simulink subsystem "Motor"  (R2024a)
settings: Solver=VariableStepAuto  StartTime=0.0  StopTime=10.0  RelTol=1e-3
values from neighbouring files (symbols this model uses):
  useGenerator = Simulink.Parameter    [LAFES_saveas.m]
settings Model: Creator=20192648  LastModifiedBy=20192648
settings ConfigComp: CovBoundaryAbsTol=1.0e-5

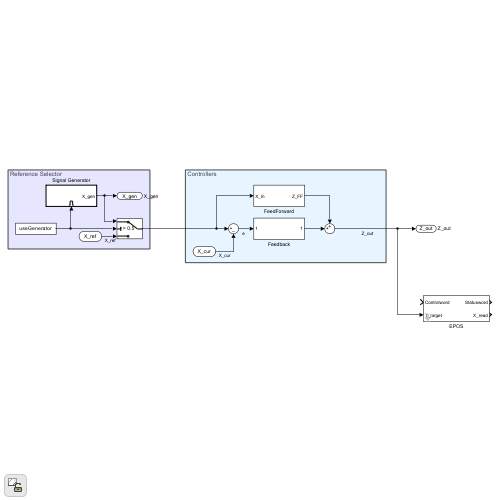
[thumbnail: Simulink's stored preview of the top-level diagram]
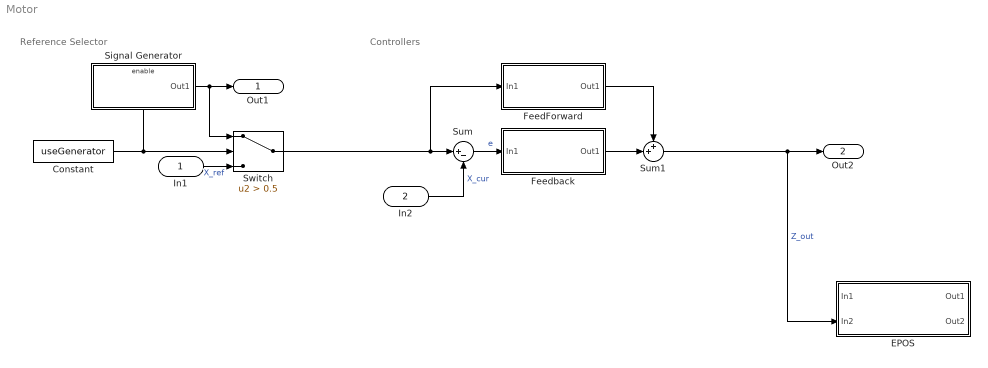
== system Motor ==
  note: Controllers
  note: Reference Selector
  In1 : Inport
  In2 : Inport  Port=2
  Constant : Constant  Value=useGenerator
  EPOS : Subsystem  mask{link_id=1, operating_mode=CyclicSynchronousTorque}
      mask prompts: link_id "link id > 0"; operating_mode "Operating mode of the drive"
      mask TypeOptions operating_mode: CyclicSynchronousPosition | CyclicSynchronousVelocity | CyclicSynchronousTorque
  FeedForward : Subsystem
  Feedback : Subsystem
  Signal Generator : Subsystem  TreatAsAtomicUnit=on
  Sum : Sum  Inputs=|+-
  Sum1 : Sum  Inputs=++|
  Switch : Switch  Criteria=u2 > Threshold  Threshold=0.5  SaturateOnIntegerOverflow=off  InputSameDT=off
  Out1 : Outport  SignalName=X_gen
  Out2 : Outport  Port=2  SignalName=Z_out
  wires:
  In2/1 -> Sum/2  "X_cur"
  Signal Generator/1(Out1) -> Out1/1, Switch/1
  Feedback/1(Out1) -> Sum1/2
  Sum/1 -> Feedback/1(In1)  "e"
  FeedForward/1(Out1) -> Sum1/1
  Sum1/1 -> Out2/1, EPOS/2(In2)  "Z_out"
  Constant/1 -> Switch/2, Signal Generator/Enable
  In1/1 -> Switch/3  "X_ref"
  Switch/1 -> Sum/1, FeedForward/1(In1)

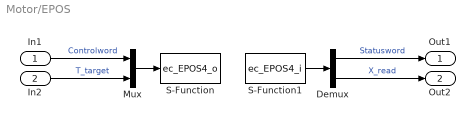
== system Motor/EPOS ==
  In1 : Inport
  In2 : Inport  Port=2
  Demux : Demux  Outputs=2
  Mux : Mux  Inputs=2
  S-Function : S-Function  FunctionName=ec_EPOS4_o  Parameters=link_id  SFunctionDeploymentMode=off  EnableBusSupport=off
  S-Function1 : S-Function  FunctionName=ec_EPOS4_i  Parameters=link_id operating_mode  SFunctionDeploymentMode=off  EnableBusSupport=off
  Out1 : Outport
  Out2 : Outport  Port=2
  wires:
  Demux/2 -> Out2/1  "X_read"
  Demux/1 -> Out1/1  "Statusword"
  S-Function1/1 -> Demux/1
  Mux/1 -> S-Function/1
  In2/1 -> Mux/2  "T_target"
  In1/1 -> Mux/1  "Controlword"

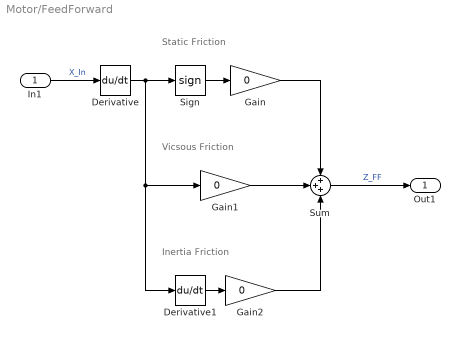
== system Motor/FeedForward ==
  note: Static Friction
  note: Vicsous Friction
  note: Inertia Friction
  In1 : Inport
  Derivative : Derivative
  Derivative1 : Derivative
  Gain : Gain  Gain=0
  Gain1 : Gain  Gain=0
  Gain2 : Gain  Gain=0
  Sign : Signum
  Sum : Sum  Inputs=+++
  Out1 : Outport
  wires:
  Sum/1 -> Out1/1  "Z_FF"
  Gain2/1 -> Sum/3
  Gain1/1 -> Sum/2
  Gain/1 -> Sum/1
  Derivative1/1 -> Gain2/1
  Derivative/1 -> Sign/1, Derivative1/1, Gain1/1
  Sign/1 -> Gain/1
  In1/1 -> Derivative/1  "X_In"

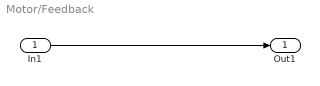
== system Motor/Feedback ==
  In1 : Inport
  Out1 : Outport
  wires:
  In1/1 -> Out1/1

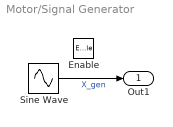
== system Motor/Signal Generator ==
  Enable : EnablePort
  Sine Wave : Sin  Amplitude=100  SampleTime=0
  Out1 : Outport
  wires:
  Sine Wave/1 -> Out1/1  "X_gen"
